simulink model "DOD"  (R2021a)
settings: Solver=VariableStepAuto  StartTime=0.0  StopTime=10.0  RelTol=1e-3
undefined symbols (not defined in the file or in its folder): C1_LUT, Capacity_LUT, cell_area, cell_Cp_heat, cell_mass, Em_LUT, h_conv, R0_LUT, R1_LUT, SOC_LUT, T_init, Temperature_LUT
settings Model: Creator=SAHIL  LastModifiedBy=SAHIL

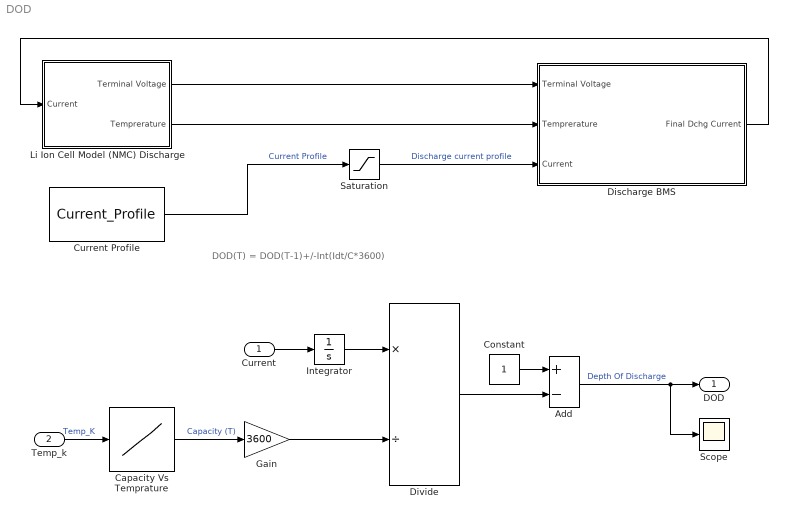
== system DOD ==
  note: DOD(T) = DOD(T-1)+/-Int(Idt/C*3600)
  Current : Inport
  Temp_k : Inport  Port=2
  Add : Sum  Inputs=+-
  Capacity Vs Temprature : Lookup_n-D  NumberOfTableDimensions=1  BreakpointsForDimension1=Temperature_LUT  Table=Capacity_LUT  InternalRulePriority=Speed  RndMeth=Simplest  InputSameDT=on
  Constant : Constant
  Current Profile : FromWorkspace  VariableName=Current_Profile
  Discharge BMS : Subsystem
  Divide : Product  Inputs=*/
  Gain : Gain  Gain=3600
  Integrator : Integrator
  Li Ion Cell Model (NMC) Discharge : Subsystem
  Saturation : Saturate  UpperLimit=inf  LowerLimit=0
  Scope : Scope
  DOD : Outport
  wires:
  Li Ion Cell Model (NMC) Discharge/2(Temprerature) -> Discharge BMS/2(Temprerature)
  Discharge BMS/1(Final Dchg Current) -> Li Ion Cell Model (NMC) Discharge/1(Current)
  Li Ion Cell Model (NMC) Discharge/1(Terminal Voltage) -> Discharge BMS/1(Terminal Voltage)
  Saturation/1 -> Discharge BMS/3(Current)  "Discharge current profile"
  Current Profile/1 -> Saturation/1  "Current Profile"
  Add/1 -> Scope/1, DOD/1  "Depth Of Discharge"
  Temp_k/1 -> Capacity Vs Temprature/1  "Temp_K"
  Gain/1 -> Divide/2
  Capacity Vs Temprature/1 -> Gain/1  "Capacity (T)"
  Divide/1 -> Add/2
  Constant/1 -> Add/1
  Current/1 -> Integrator/1
  Integrator/1 -> Divide/1

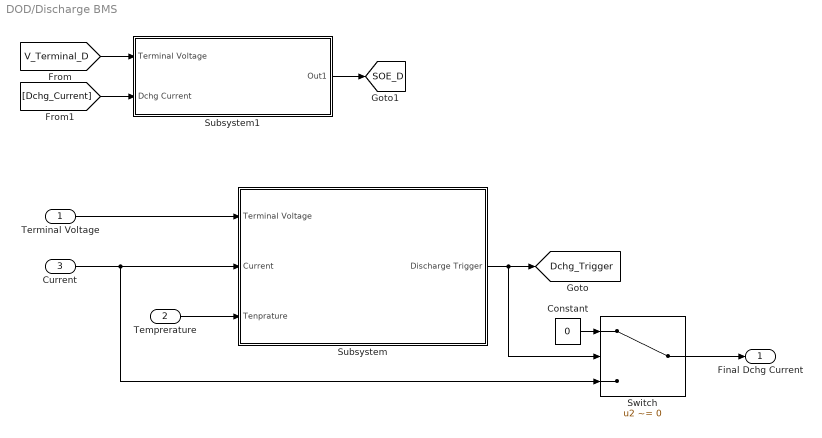
== system DOD/Discharge BMS ==
  Terminal Voltage : Inport
  Temprerature : Inport  Port=2
  Current : Inport  Port=3
  Constant : Constant  Value=0
  Subsystem : Subsystem
  Subsystem1 : Subsystem
  Switch : Switch  Criteria=u2 ~= 0
  Final Dchg Current : Outport
  tag scope: Dchg_Trigger=global, SOE_D=global
  wires:
  Terminal Voltage/1 -> Subsystem/1(Terminal Voltage)
  Current/1 -> Switch/3, Subsystem/2(Current)
  Temprerature/1 -> Subsystem/3(Tenprature)
  Subsystem/1(Discharge Trigger) -> Switch/2, [Dchg_Trigger]
  Constant/1 -> Switch/1
  Switch/1 -> Final Dchg Current/1
  Subsystem1/1(Out1) -> [SOE_D]
  [V_Terminal_D] -> Subsystem1/1(Terminal Voltage)
  [Dchg_Current] -> Subsystem1/2(Dchg Current)

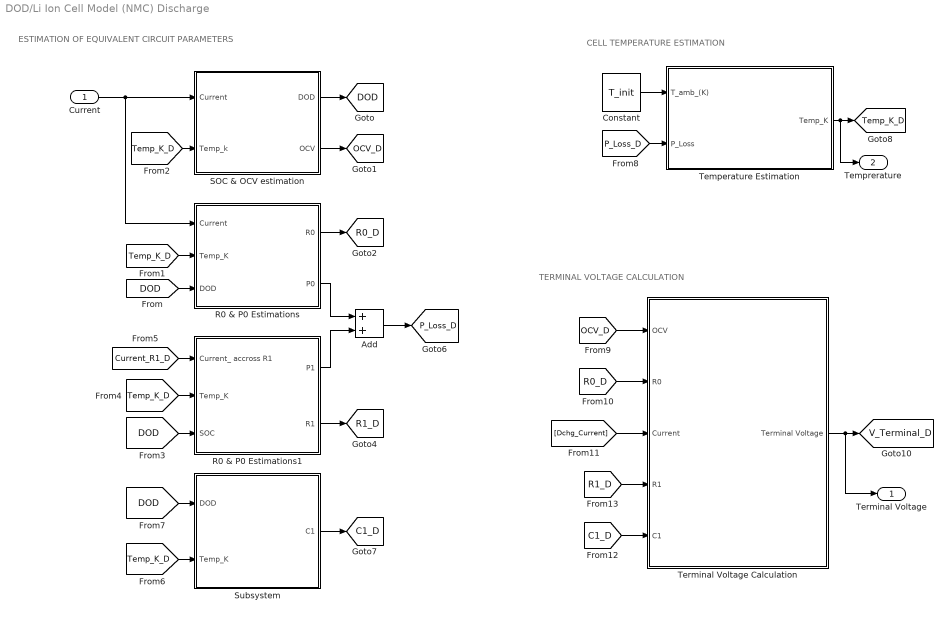
== system DOD/Li Ion Cell Model (NMC) Discharge ==
  note: TERMINAL VOLTAGE CALCULATION
  note: CELL TEMPERATURE ESTIMATION
  note: ESTIMATION OF EQUIVALENT CIRCUIT PARAMETERS
  Current : Inport
  Add : Sum
  Constant : Constant  Value=T_init
  R0 & P0 Estimations : Subsystem
  R0 & P0 Estimations1 : Subsystem
  SOC & OCV estimation : Subsystem
  Subsystem : Subsystem
  Temperature Estimation : Subsystem
  Terminal Voltage Calculation : Subsystem
  Terminal Voltage : Outport
  Temprerature : Outport  Port=2
  tag scope: C1_D=global, DOD=global, OCV_D=global, P_Loss_D=global, R0_D=global, R1_D=global, Temp_K_D=global, V_Terminal_D=global
  wires:
  Current/1 -> R0 & P0 Estimations/1(Current), SOC & OCV estimation/1(Current)
  [Temp_K_D] -> SOC & OCV estimation/2(Temp_k)
  SOC & OCV estimation/1(DOD) -> [DOD]
  SOC & OCV estimation/2(OCV) -> [OCV_D]
  [DOD] -> R0 & P0 Estimations/3(DOD)
  [Temp_K_D] -> R0 & P0 Estimations/2(Temp_K)
  R0 & P0 Estimations/1(R0) -> [R0_D]
  R0 & P0 Estimations/2(P0) -> Add/1
  [DOD] -> R0 & P0 Estimations1/3(SOC)
  [Temp_K_D] -> R0 & P0 Estimations1/2(Temp_K)
  [Current_R1_D] -> R0 & P0 Estimations1/1(Current_ accross R1)
  R0 & P0 Estimations1/1(P1) -> Add/2
  Add/1 -> [P_Loss_D]
  R0 & P0 Estimations1/2(R1) -> [R1_D]
  Subsystem/1(C1) -> [C1_D]
  Temperature Estimation/1(Temp_K) -> Temprerature/1, [Temp_K_D]
  Constant/1 -> Temperature Estimation/1(T_amb_(K))
  [P_Loss_D] -> Temperature Estimation/2(P_Loss)
  [OCV_D] -> Terminal Voltage Calculation/1(OCV)
  [R0_D] -> Terminal Voltage Calculation/2(R0)
  [Dchg_Current] -> Terminal Voltage Calculation/3(Current)
  Terminal Voltage Calculation/1(Terminal Voltage) -> Terminal Voltage/1, [V_Terminal_D]
  [DOD] -> Subsystem/1(DOD)
  [Temp_K_D] -> Subsystem/2(Temp_K)
  [R1_D] -> Terminal Voltage Calculation/4(R1)
  [C1_D] -> Terminal Voltage Calculation/5(C1)

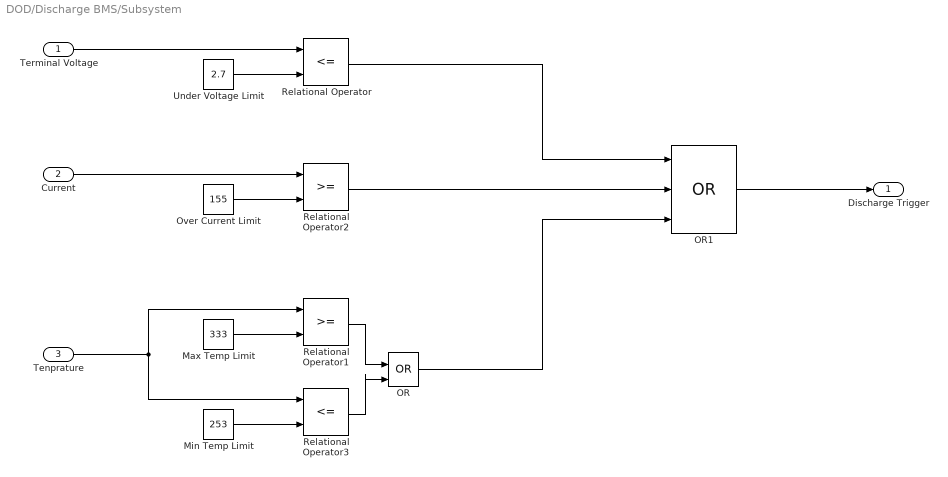
== system DOD/Discharge BMS/Subsystem ==
  Terminal Voltage : Inport
  Current : Inport  Port=2
  Tenprature : Inport  Port=3
  Max Temp Limit : Constant  Value=333
  Min Temp Limit : Constant  Value=253
  OR : Logic  Operator=OR  IconShape=distinctive  AllPortsSameDT=off  OutDataTypeStr=boolean
  OR1 : Logic  Operator=OR  Inputs=3  IconShape=distinctive  AllPortsSameDT=off  OutDataTypeStr=boolean
  Over Current Limit : Constant  Value=155
  Relational Operator : RelationalOperator  Operator=<=  OutDataTypeStr=boolean  RndMeth=Simplest
  Relational Operator1 : RelationalOperator  OutDataTypeStr=boolean  RndMeth=Simplest
  Relational Operator2 : RelationalOperator  OutDataTypeStr=boolean  RndMeth=Simplest
  Relational Operator3 : RelationalOperator  Operator=<=  OutDataTypeStr=boolean  RndMeth=Simplest
  Under Voltage Limit : Constant  Value=2.7
  Discharge Trigger : Outport
  wires:
  Min Temp Limit/1 -> Relational Operator3/2
  OR/1 -> OR1/3
  Relational Operator1/1 -> OR/1
  Max Temp Limit/1 -> Relational Operator1/2
  Tenprature/1 -> Relational Operator3/1, Relational Operator1/1
  Relational Operator2/1 -> OR1/2
  Relational Operator/1 -> OR1/1
  Over Current Limit/1 -> Relational Operator2/2
  Under Voltage Limit/1 -> Relational Operator/2
  Relational Operator3/1 -> OR/2
  OR1/1 -> Discharge Trigger/1
  Current/1 -> Relational Operator2/1
  Terminal Voltage/1 -> Relational Operator/1

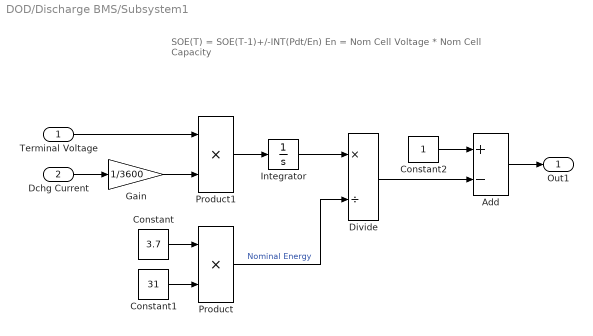
== system DOD/Discharge BMS/Subsystem1 ==
  note: SOE(T) = SOE(T-1)+/-INT(Pdt/En)
      | En = Nom Cell Voltage * Nom Cell Capacity
  Terminal Voltage : Inport
  Dchg Current : Inport  Port=2
  Add : Sum  Inputs=+-
  Constant : Constant  Value=3.7
  Constant1 : Constant  Value=31
  Constant2 : Constant
  Divide : Product  Inputs=*/
  Gain : Gain  Gain=1/3600
  Integrator : Integrator
  Product : Product
  Product1 : Product
  Out1 : Outport
  wires:
  Constant/1 -> Product/1
  Constant1/1 -> Product/2
  Product/1 -> Divide/2  "Nominal Energy"
  Dchg Current/1 -> Gain/1
  Gain/1 -> Product1/2
  Terminal Voltage/1 -> Product1/1
  Product1/1 -> Integrator/1
  Integrator/1 -> Divide/1
  Constant2/1 -> Add/1
  Divide/1 -> Add/2
  Add/1 -> Out1/1

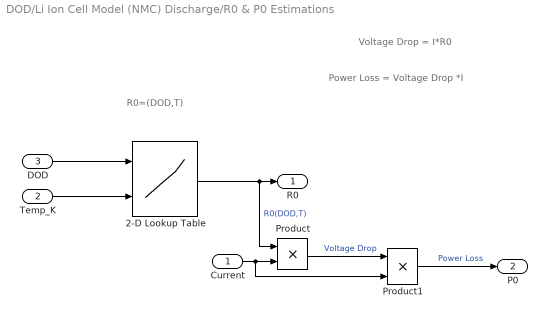
== system DOD/Li Ion Cell Model (NMC) Discharge/R0 & P0 Estimations ==
  note: Power Loss = Voltage Drop *I
  note: Voltage Drop = I*R0
  note: R0=(DOD,T)
  Current : Inport
  Temp_K : Inport  Port=2
  DOD : Inport  Port=3
  2-D Lookup Table : Lookup_n-D  BreakpointsForDimension1=SOC_LUT  BreakpointsForDimension2=Temperature_LUT  Table=R0_LUT  InternalRulePriority=Speed  RndMeth=Simplest  InputSameDT=on
      settings: InputPortMap=u0,u1
  Product : Product
  Product1 : Product
  R0 : Outport
  P0 : Outport  Port=2
  wires:
  DOD/1 -> 2-D Lookup Table/1
  Temp_K/1 -> 2-D Lookup Table/2
  2-D Lookup Table/1 -> Product/1, R0/1  "R0(DOD,T)"
  Current/1 -> Product1/2, Product/2
  Product/1 -> Product1/1  "Voltage Drop"
  Product1/1 -> P0/1  "Power Loss"

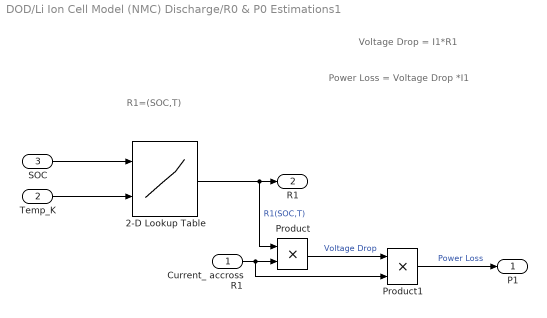
== system DOD/Li Ion Cell Model (NMC) Discharge/R0 & P0 Estimations1 ==
  note: Power Loss = Voltage Drop *I1
  note: Voltage Drop = I1*R1
  note: R1=(SOC,T)
  Current_ accross R1 : Inport
  Temp_K : Inport  Port=2
  SOC : Inport  Port=3
  2-D Lookup Table : Lookup_n-D  BreakpointsForDimension1=SOC_LUT  BreakpointsForDimension2=Temperature_LUT  Table=R1_LUT  InternalRulePriority=Speed  RndMeth=Simplest  InputSameDT=on
      settings: InputPortMap=u0,u1
  Product : Product
  Product1 : Product
  P1 : Outport
  R1 : Outport  Port=2
  wires:
  SOC/1 -> 2-D Lookup Table/1
  Temp_K/1 -> 2-D Lookup Table/2
  2-D Lookup Table/1 -> Product/1, R1/1  "R1(SOC,T)"
  Current_ accross R1/1 -> Product1/2, Product/2
  Product/1 -> Product1/1  "Voltage Drop"
  Product1/1 -> P1/1  "Power Loss"

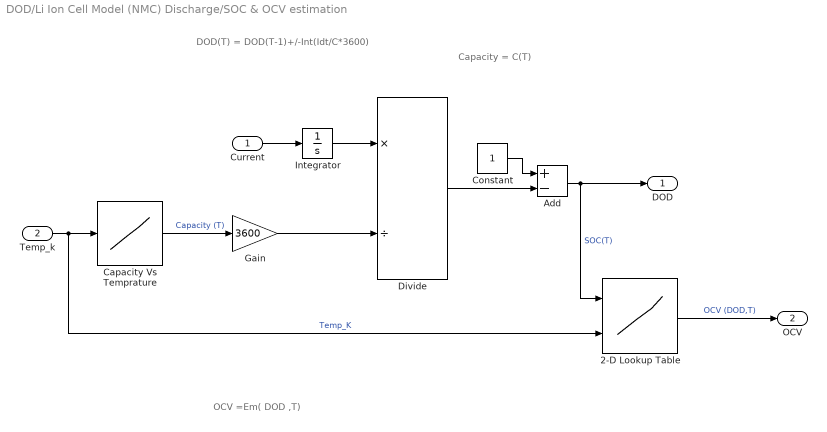
== system DOD/Li Ion Cell Model (NMC) Discharge/SOC & OCV estimation ==
  note: OCV =Em( DOD ,T)
  note: Capacity = C(T)
  note: DOD(T) = DOD(T-1)+/-Int(Idt/C*3600)
  Current : Inport
  Temp_k : Inport  Port=2
  2-D Lookup Table : Lookup_n-D  BreakpointsForDimension1=SOC_LUT  BreakpointsForDimension2=Temperature_LUT  Table=Em_LUT  InternalRulePriority=Speed  RndMeth=Simplest  InputSameDT=on
      settings: InputPortMap=u0,u1
  Add : Sum  Inputs=+-
  Capacity Vs Temprature : Lookup_n-D  NumberOfTableDimensions=1  BreakpointsForDimension1=Temperature_LUT  Table=Capacity_LUT  InternalRulePriority=Speed  RndMeth=Simplest  InputSameDT=on
  Constant : Constant
  Divide : Product  Inputs=*/
  Gain : Gain  Gain=3600
  Integrator : Integrator
  DOD : Outport
  OCV : Outport  Port=2
  wires:
  Temp_k/1 -> 2-D Lookup Table/2, Capacity Vs Temprature/1  "Temp_K"
  Capacity Vs Temprature/1 -> Gain/1  "Capacity (T)"
  Current/1 -> Integrator/1
  Integrator/1 -> Divide/1
  Gain/1 -> Divide/2
  Divide/1 -> Add/2
  Constant/1 -> Add/1
  Add/1 -> 2-D Lookup Table/1, DOD/1  "SOC(T)"
  2-D Lookup Table/1 -> OCV/1  "OCV (DOD,T)"

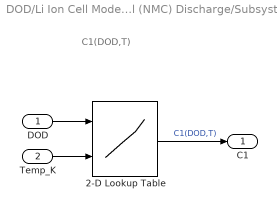
== system DOD/Li Ion Cell Model (NMC) Discharge/Subsystem ==
  note: C1(DOD,T)
  DOD : Inport
  Temp_K : Inport  Port=2
  2-D Lookup Table : Lookup_n-D  BreakpointsForDimension1=SOC_LUT  BreakpointsForDimension2=Temperature_LUT  Table=C1_LUT  InternalRulePriority=Speed  RndMeth=Simplest  InputSameDT=on
      settings: InputPortMap=u0,u1
  C1 : Outport
  wires:
  DOD/1 -> 2-D Lookup Table/1
  Temp_K/1 -> 2-D Lookup Table/2
  2-D Lookup Table/1 -> C1/1  "C1(DOD,T)"

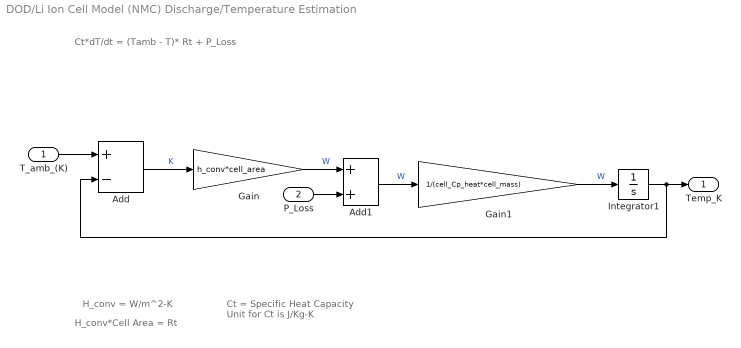
== system DOD/Li Ion Cell Model (NMC) Discharge/Temperature Estimation ==
  note: Ct = Specific Heat Capacity
      | Unit for Ct is J/Kg-K
  note: H_conv*Cell Area = Rt
  note: H_conv = W/m^2-K
  note: Ct*dT/dt = (Tamb - T)* Rt + P_Loss
  T_amb_(K) : Inport
  P_Loss : Inport  Port=2
  Add : Sum  Inputs=+-
  Add1 : Sum
  Gain : Gain  Gain=h_conv*cell_area
  Gain1 : Gain  Gain=1/(cell_Cp_heat*cell_mass)
  Integrator1 : Integrator  InitialCondition=293.15
  Temp_K : Outport
  wires:
  T_amb_(K)/1 -> Add/1
  Add/1 -> Gain/1  "K"
  Gain/1 -> Add1/1  "W"
  P_Loss/1 -> Add1/2
  Add1/1 -> Gain1/1  "W"
  Gain1/1 -> Integrator1/1  "W"
  Integrator1/1 -> Add/2, Temp_K/1

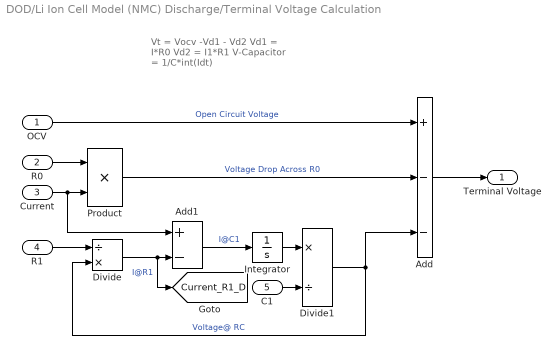
== system DOD/Li Ion Cell Model (NMC) Discharge/Terminal Voltage Calculation ==
  note: Vt = Vocv -Vd1 - Vd2
      | Vd1 = I*R0
      | Vd2 = I1*R1
      | V-Capacitor = 1/C*int(Idt)
  OCV : Inport
  R0 : Inport  Port=2
  Current : Inport  Port=3
  R1 : Inport  Port=4
  C1 : Inport  Port=5
  Add : Sum  Inputs=+--
  Add1 : Sum  Inputs=+-
  Divide : Product  Inputs=/*
  Divide1 : Product  Inputs=*/
  Integrator : Integrator
  Product : Product
  Terminal Voltage : Outport
  tag scope: Current_R1_D=global
  wires:
  OCV/1 -> Add/1  "Open Circuit Voltage"
  Add/1 -> Terminal Voltage/1
  R0/1 -> Product/1
  Current/1 -> Add1/1, Product/2
  Product/1 -> Add/2  "Voltage Drop Across R0"
  R1/1 -> Divide/1
  Divide/1 -> Add1/2, [Current_R1_D]  "I@R1"
  Add1/1 -> Integrator/1  "I@C1"
  C1/1 -> Divide1/2
  Integrator/1 -> Divide1/1
  Divide1/1 -> Divide/2, Add/3  "Voltage@ RC"
